simulink model "Attitude_Control_2nd_Linear_ADRC_Simulink"  (R2016b)
settings: Solver=VariableStepAuto  StartTime=0.0  StopTime=20  RelTol=1e-3
values from neighbouring files (symbols this model uses):
  b_0 = 0.04    [Attitude_Control_2nd_Linear_ADRC.m]
  b_0_p = 0.4    [Attitude_Control_2nd_Linear_ADRC.m]
  b_0_r = 0.4    [Attitude_Control_2nd_Linear_ADRC.m]
  b_0_y = 0.04    [Attitude_Control_2nd_Linear_ADRC.m]
  beta_01 = 30    [Attitude_Control_2nd_Linear_ADRC.m]
  beta_01_p = 30    [Attitude_Control_2nd_Linear_ADRC.m]
  beta_01_r = 30    [Attitude_Control_2nd_Linear_ADRC.m]
  beta_01_y = 30    [Attitude_Control_2nd_Linear_ADRC.m]
  beta_02 = 300    [Attitude_Control_2nd_Linear_ADRC.m]
  beta_02_p = 300    [Attitude_Control_2nd_Linear_ADRC.m]
  beta_02_r = 300    [Attitude_Control_2nd_Linear_ADRC.m]
  beta_02_y = 300    [Attitude_Control_2nd_Linear_ADRC.m]
  beta_03 = 1000    [Attitude_Control_2nd_Linear_ADRC.m]
  beta_03_p = 1000    [Attitude_Control_2nd_Linear_ADRC.m]
  beta_03_r = 1000    [Attitude_Control_2nd_Linear_ADRC.m]
  beta_03_y = 1000    [Attitude_Control_2nd_Linear_ADRC.m]
  beta_1 = 200    [Attitude_Control_2nd_Linear_ADRC.m]
  beta_1_p = 200    [Attitude_Control_2nd_Linear_ADRC.m]
  beta_1_r = 200    [Attitude_Control_2nd_Linear_ADRC.m]
  beta_1_y = 200    [Attitude_Control_2nd_Linear_ADRC.m]
  beta_2 = 120    [Attitude_Control_2nd_Linear_ADRC.m]
  beta_2_p = 120    [Attitude_Control_2nd_Linear_ADRC.m]
  beta_2_r = 120    [Attitude_Control_2nd_Linear_ADRC.m]
  beta_2_y = 120    [Attitude_Control_2nd_Linear_ADRC.m]
  fp = 1e3    (= 1000)    [Attitude_Control_2nd_Linear_ADRC.m]
libraries: simulink x1
settings Model: Creator=admin  LastModifiedBy=admin

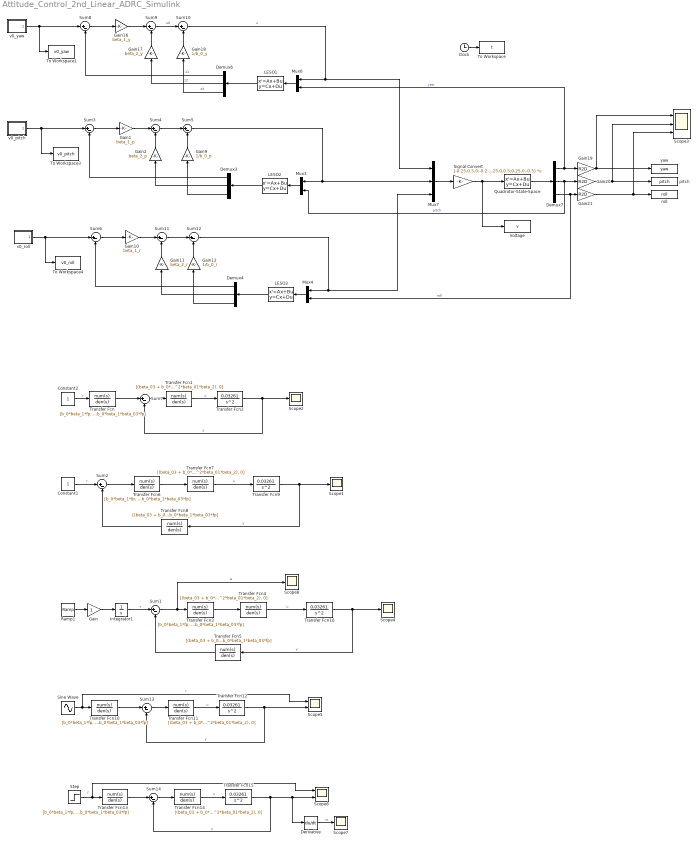
== system Attitude_Control_2nd_Linear_ADRC_Simulink ==
  note: r
  Clock : Clock
  Constant1 : Constant
      mask Display: disp('in')
  Constant2 : Constant
      mask Display: disp('in')
  Demux{3..4,6..7} (4 alike) : Demux  Outputs=3
  Derivative : Derivative
  Gain : Gain
  Gain1 : Gain  Gain=beta_1_p
      mask Display: disp('\beta_{1p}','texmode','on')
  Gain10 : Gain  Gain=beta_1_r
      mask Display: disp('\beta_{1r}','texmode','on')
  Gain11 : Gain  Gain=beta_2_r
      mask Display: disp('\beta_{2r}','texmode','on')
  Gain12 : Gain  Gain=1/b_0_r
      mask Display: disp('1/b_{0r}','texmode','on')
  Gain16 : Gain  Gain=beta_1_y
      mask Display: disp('\beta_{1y}','texmode','on')
  Gain17 : Gain  Gain=beta_2_y
      mask Display: disp('\beta_{2y}','texmode','on')
  Gain18 : Gain  Gain=1/b_0_y
      mask Display: disp('1/b_{0y}','texmode','on')
  Gain19 : Gain  Gain=R2D  mask{R2D=180/pi}
  Gain2 : Gain  Gain=beta_2_p
      mask Display: disp('\beta_{2p}','texmode','on')
  Gain20 : Gain  Gain=R2D  mask{R2D=180/pi}
  Gain21 : Gain  Gain=R2D  mask{R2D=180/pi}
  Gain9 : Gain  Gain=1/b_0_p
      mask Display: disp('1/b_{0p}','texmode','on')
  Integrator1 : Integrator
  LESO1 : StateSpace  A=[-beta_01_y 1 0;-beta_02_y 0 1;-beta_03_y 0 0]  B=[0 beta_01_y;b_0_y beta_02_y;0 beta_03_y]  C=[1 0 0;0 1 0;0 0 1]  D=[0 0;0 0;0 0]  X0=0
  LESO2 : StateSpace  A=[-beta_01_p 1 0;-beta_02_p 0 1;-beta_03_p 0 0]  B=[0 beta_01_p;b_0_p beta_02_p;0 beta_03_p]  C=[1 0 0;0 1 0;0 0 1]  D=[0 0;0 0;0 0]  X0=0
  LESO3 : StateSpace  A=[-beta_01_r 1 0;-beta_02_r 0 1;-beta_03_r 0 0]  B=[0 beta_01_r;b_0_r beta_02_r;0 beta_03_r]  C=[1 0 0;0 1 0;0 0 1]  D=[0 0;0 0;0 0]  X0=0
  Mux3 : Mux  Inputs=2
  Mux4 : Mux  Inputs=2
  Mux6 : Mux  Inputs=2
  Mux7 : Mux  Inputs=3
  Quadrotor-State-Space : StateSpace  A=[0,0,0,1,0,0;0,0,0,0,1,0;0,0,0,0,0,1;0,0,0,0,0,0;0,0,0,0,0,0;0,0,0,0,0,0]  B=[0,0,0,0;0,0,0,0;0,0,0,0;k_tc/J_y,k_tc/J_y,k_tn/J_y,k_tn/J_y;l*k_f/J_p,-l*k_f/J_p,0,0;0,0,l*k_f/J_r,-l*k_f/J_r]  C=[1,0,0,0,0,0;0,1,0,0,0,0;0,0,1,0,0,0]  D=[0,0,0,0;0,0,0,0;0,0,0,0]  X0=[0;0;0;0;0;0]  mask{k_tn=0.0036, k_tc=-0.0036, k_f=0.1188, J_y=0.1104, J_p=0.0552, J_r=0.0552, l=0.197}
      mask prompts: k_tn "k_tn 顺时针螺旋桨推力矩系数(N·m/V)"; k_tc "k_tc 逆时针螺旋桨推力矩系数(N·m/V)"; k_f "k_f 螺旋桨推力系数(N/V)"; J_y "J_y 偏航轴转动惯量(kg·m²)"; J_p "J_p 俯仰轴转动惯量(kg·m²)"; J_r "J_r 滚转轴转动惯量(kg·m²)"; l "l 旋转中心到螺旋桨中心的距离(m)"
  Ramp1 : simulink/Sources/Ramp  slope=1  start=0  X0=0
  Scope{1..2,4,7..8} (5 alike) : Scope
  Scope3 : Scope  NumInputPorts=3
  Scope5 : Scope  NumInputPorts=2
  Scope6 : Scope  NumInputPorts=2
  Signal Convert : Gain  Gain=[-0.25,0.5,0;-0.25,-0.5,0;0.25,0,0.5;0.25,0,-0.5]  Multiplication=Matrix(K*u)
  Sine Wave : Sin  Amplitude=3*pi/180  SampleTime=0
  Step : Step  After=30*pi/180  SampleTime=0
  Sum{1..14} (14 alike) : Sum  Inputs=|+-
  To Workspace : ToWorkspace  VariableName=t  SampleTime=-1
  To Workspace1 : ToWorkspace  VariableName=v0_yaw  SampleTime=-1
  To Workspace3 : ToWorkspace  VariableName=v0_pitch  SampleTime=-1
  To Workspace4 : ToWorkspace  VariableName=v0_roll  SampleTime=-1
  Transfer Fcn{,3,6,10,13} (5 alike) : TransferFcn  Numerator=[b_0*beta_1*fp, b_0*beta_01*beta_1*fp, b_0*beta_1*beta_02*fp, b_0*beta_1*beta_03*fp]  Denominator=[(beta_03 + b_0*beta_01*beta_1 + b_0*beta_02*beta_2), (beta_03*fp + b_0*beta_1*beta_02 + b_0*beta_2*beta_03 + b_0*beta_01*beta_1*fp + b_0*beta_02*beta_2*fp), (b_0*beta_1*beta_03 + b_0*beta_1*beta_02*fp + b_0*beta_2*beta_03*fp), b_0*beta_1*beta_03*fp]
      mask Display: disp('C_{11}(s)','texmode','on')
  Transfer Fcn{1,4,7,11,14} (5 alike) : TransferFcn  Numerator=[(beta_03 + b_0*beta_01*beta_1 + b_0*beta_02*beta_2), (b_0*beta_1*beta_02 + b_0*beta_2*beta_03), b_0*beta_1*beta_03]  Denominator=[b_0, (beta_2*b_0^2 + beta_01*b_0), (b_0*beta_02 + b_0^2*beta_1 + b_0^2*beta_01*beta_2), 0]
      mask Display: disp('C_{2}(s)','texmode','on')
  Transfer Fcn{2,9,12,15..16} (5 alike) : TransferFcn  Numerator=[0.03261]  Denominator=[1 0 0]
      mask Display: disp('G(s)')
  Transfer Fcn5 : TransferFcn  Numerator=[(beta_03 + b_0*beta_01*beta_1 + b_0*beta_02*beta_2), (beta_03*fp + b_0*beta_1*beta_02 + b_0*beta_2*beta_03 + b_0*beta_01*beta_1*fp + b_0*beta_02*beta_2*fp), (b_0*beta_1*beta_03 + b_0*beta_1*beta_02*fp + b_0*beta_2*beta_03*fp), b_0*beta_1*beta_03*fp]  Denominator=[b_0*beta_1*fp, b_0*beta_01*beta_1*fp, b_0*beta_1*beta_02*fp, b_0*beta_1*beta_03*fp]
      mask Display: disp('1/C_{11}(s)','texmode','on')
  Transfer Fcn8 : TransferFcn  Numerator=[(beta_03 + b_0*beta_01*beta_1 + b_0*beta_02*beta_2), (beta_03*fp + b_0*beta_1*beta_02 + b_0*beta_2*beta_03 + b_0*beta_01*beta_1*fp + b_0*beta_02*beta_2*fp), (b_0*beta_1*beta_03 + b_0*beta_1*beta_02*fp + b_0*beta_2*beta_03*fp), b_0*beta_1*beta_03*fp]  Denominator=[b_0*beta_1*fp, b_0*beta_01*beta_1*fp, b_0*beta_1*beta_02*fp, b_0*beta_1*beta_03*fp]
      mask Display: disp('1/C_{11}(s)','texmode','on')
  Voltage : ToWorkspace  VariableName=v  SampleTime=-1
  pitch : ToWorkspace  VariableName=pitch  SampleTime=-1
  roll : ToWorkspace  VariableName=roll  SampleTime=-1
  v0_pitch : Subsystem
  v0_roll : Subsystem
  v0_yaw : Subsystem
  yaw : ToWorkspace  VariableName=yaw  SampleTime=-1
  wires:
  Transfer Fcn1/1 -> Transfer Fcn2/1  "u"
  Sum7/1 -> Transfer Fcn1/1
  LESO1/1 -> Demux6/1
  Demux6/1 -> Sum8/2  "z1"
  Demux6/2 -> Gain17/1  "z2"
  Gain17/1 -> Sum9/2
  Gain16/1 -> Sum9/1
  Demux6/3 -> Gain18/1  "z3"
  Sum9/1 -> Sum10/1  "u0"
  Sum8/1 -> Gain16/1
  Gain18/1 -> Sum10/2
  Sum10/1 -> Mux7/1, Mux6/1  "u"
  Mux6/1 -> LESO1/1
  v0_yaw/1(v0_yaw) -> To Workspace1/1, Sum8/1
  Mux7/1 -> Signal Convert/1
  Signal Convert/1 -> Voltage/1, Quadrotor-State-Space/1
  Quadrotor-State-Space/1 -> Demux7/1
  Gain19/1 -> Scope3/1, yaw/1
  Gain20/1 -> Scope3/2, pitch/1
  Gain21/1 -> Scope3/3, roll/1
  Demux7/2 -> Mux3/2, Gain20/1  "pitch"
  Demux7/1 -> Mux6/2, Gain19/1  "yaw"
  Demux7/3 -> Mux4/2, Gain21/1  "roll"
  Transfer Fcn6/1 -> Transfer Fcn7/1
  Transfer Fcn7/1 -> Transfer Fcn9/1  "u"
  Transfer Fcn8/1 -> Sum2/2
  Sum2/1 -> Transfer Fcn6/1
  Constant1/1 -> Sum2/1  "r"
  Transfer Fcn9/1 -> Scope1/1, Transfer Fcn8/1  "y"
  Transfer Fcn/1 -> Sum7/1
  Transfer Fcn2/1 -> Scope2/1, Sum7/2  "y"
  LESO2/1 -> Demux3/1
  Demux3/1 -> Sum3/2
  Demux3/2 -> Gain2/1
  Gain2/1 -> Sum4/2
  Gain1/1 -> Sum4/1
  Demux3/3 -> Gain9/1
  Sum4/1 -> Sum5/1
  Sum3/1 -> Gain1/1
  Gain9/1 -> Sum5/2
  Sum5/1 -> Mux3/1, Mux7/2
  Mux3/1 -> LESO2/1
  v0_pitch/1(v0_pitch) -> To Workspace3/1, Sum3/1
  LESO3/1 -> Demux4/1
  Demux4/1 -> Sum6/2
  Demux4/2 -> Gain11/1
  Gain11/1 -> Sum11/2
  Gain10/1 -> Sum11/1
  Demux4/3 -> Gain12/1
  Sum11/1 -> Sum12/1
  Sum6/1 -> Gain10/1
  Gain12/1 -> Sum12/2
  Sum12/1 -> Mux7/3, Mux4/1
  Mux4/1 -> LESO3/1
  v0_roll/1(v0_roll) -> To Workspace4/1, Sum6/1
  Clock/1 -> To Workspace/1
  Ramp1/1 -> Gain/1
  Constant2/1 -> Transfer Fcn/1  "r"
  Gain/1 -> Integrator1/1
  Transfer Fcn11/1 -> Transfer Fcn12/1  "u"
  Sum13/1 -> Transfer Fcn11/1
  Transfer Fcn10/1 -> Sum13/1
  Transfer Fcn12/1 -> Scope5/2, Sum13/2  "y"
  Sine Wave/1 -> Scope5/1, Transfer Fcn10/1  "r"
  Transfer Fcn14/1 -> Transfer Fcn15/1  "u"
  Sum14/1 -> Transfer Fcn14/1
  Transfer Fcn13/1 -> Sum14/1
  Transfer Fcn15/1 -> Derivative/1, Scope6/2, Sum14/2  "y"
  Step/1 -> Scope6/1, Transfer Fcn13/1
  Derivative/1 -> Scope7/1  "w"
  Transfer Fcn3/1 -> Transfer Fcn4/1
  Transfer Fcn4/1 -> Transfer Fcn16/1  "u"
  Transfer Fcn5/1 -> Sum1/2
  Sum1/1 -> Scope8/1, Transfer Fcn3/1  "e"
  Integrator1/1 -> Sum1/1  "r"
  Transfer Fcn16/1 -> Scope4/1, Transfer Fcn5/1  "y"

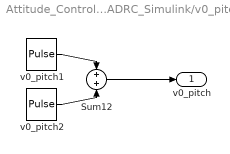
== system Attitude_Control_2nd_Linear_ADRC_Simulink/v0_pitch ==
  Sum12 : Sum
  v0_pitch1 : DiscretePulseGenerator  PulseType=Time based  Amplitude=3*pi/180  Period=10  PulseWidth=50  PhaseDelay=5
  v0_pitch2 : DiscretePulseGenerator  PulseType=Time based  Amplitude=-3*pi/180  Period=10  PulseWidth=50
  v0_pitch : Outport
  wires:
  v0_pitch2/1 -> Sum12/2
  Sum12/1 -> v0_pitch/1
  v0_pitch1/1 -> Sum12/1

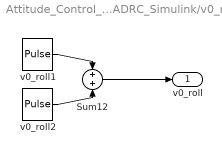
== system Attitude_Control_2nd_Linear_ADRC_Simulink/v0_roll ==
  Sum12 : Sum
  v0_roll1 : DiscretePulseGenerator  PulseType=Time based  Amplitude=3*pi/180  Period=10  PulseWidth=50  PhaseDelay=5
  v0_roll2 : DiscretePulseGenerator  PulseType=Time based  Amplitude=-3*pi/180  Period=10  PulseWidth=50
  v0_roll : Outport
  wires:
  v0_roll2/1 -> Sum12/2
  Sum12/1 -> v0_roll/1
  v0_roll1/1 -> Sum12/1

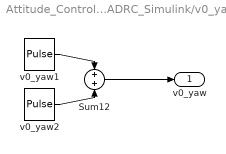
== system Attitude_Control_2nd_Linear_ADRC_Simulink/v0_yaw ==
  Sum12 : Sum
  v0_yaw1 : DiscretePulseGenerator  PulseType=Time based  Amplitude=3*pi/180  Period=10  PulseWidth=50  PhaseDelay=5
  v0_yaw2 : DiscretePulseGenerator  PulseType=Time based  Amplitude=-3*pi/180  Period=10  PulseWidth=50
  v0_yaw : Outport
  wires:
  v0_yaw2/1 -> Sum12/2
  Sum12/1 -> v0_yaw/1
  v0_yaw1/1 -> Sum12/1
